simulink model "test_quadrotor_design"  (R2021a)
settings: Solver=VariableStepAuto  StartTime=0.0  StopTime=10.0  RelTol=1e-3
values from neighbouring files (symbols this model uses):
  S = [S1;zeros(6,4)]    [get_closed_loop_quadrotor.m]
libraries: cstblocks x2
settings Model: Creator=adwai  LastModifiedBy=adwai

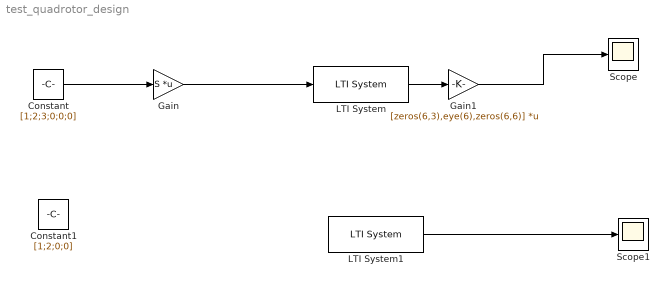
== system test_quadrotor_design ==
  Constant : Constant  Value=[1;2;3;0;0;0]
  Constant1 : Constant  Value=[1;2;0;0]
  Gain : Gain  Gain=S  Multiplication=Matrix(K*u)
  Gain1 : Gain  Gain=[zeros(6,3),eye(6),zeros(6,6)]  Multiplication=Matrix(K*u)
  LTI System : cstblocks/LTI System  sys=G_cl  IC=[]
  LTI System1 : cstblocks/LTI System  sys=G_quad_cl  IC=[]
  Scope : Scope
  Scope1 : Scope
  wires:
  Gain/1 -> LTI System/1
  Constant/1 -> Gain/1
  LTI System/1 -> Gain1/1
  Gain1/1 -> Scope/1
  LTI System1/1 -> Scope1/1
